simulink model "untitled"  (R2022a)
settings: Solver=FixedStepAuto  StartTime=0.0  StopTime=50  FixedStep=0.0001  RelTol=1e-3
PreLoadFcn:
  | % FK=ss(A,B,C,D);
  | % FK1=tf(FK)
  | G2=tf([-253.6 -141.7 -700.8 2.288],[1 6.083 7.223 17.36 0.6782]);
  | G=G2;
  | figure
  | rlocus(G)
  | rlocfind(G)
  | KP=0.0213;
  | load('peiping.mat');
model workspace: external: MAT-File D:\Desktop\无人机双环pid\peiping.mat (data not in the file)
values from neighbouring files (symbols this model uses):
  A = [0 0 0 0 9.794 0 0 -3.5879 0 0 0 0 ... (144 elements, 12x12)]    [peiping.mat]
  B = [0 0 0 0.0146 0 -0.271 0 0 0 0 -0.151 0 ... (48 elements, 12x4)]    [peiping.mat]
  C = [0 -2 0 0 0 0 -3.5879 0 0 57.3 0 0 ... (240 elements, 20x12)]    [peiping.mat]
  D = [0 0 0 0 0 0 0 0 0 0 0 0 ... (80 elements, 20x4)]    [peiping.mat]
libraries: slpidlib x9
settings Model: PacingRate=1000  Creator=yuhangmeng  LastModifiedBy=yuhangmeng
settings SolverCC: ZeroCrossAlgorithm=Adaptive
settings DataIOCC: ExternalInput=getinputstruct(op_trim2)  InitialState=getstatestruct(op_trim2)
settings DebuggingCC: IgnoredZcDiagnostic=none

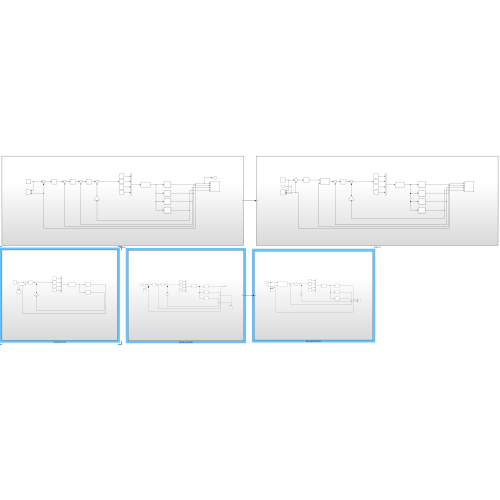
[thumbnail: Simulink's stored preview of the top-level diagram]
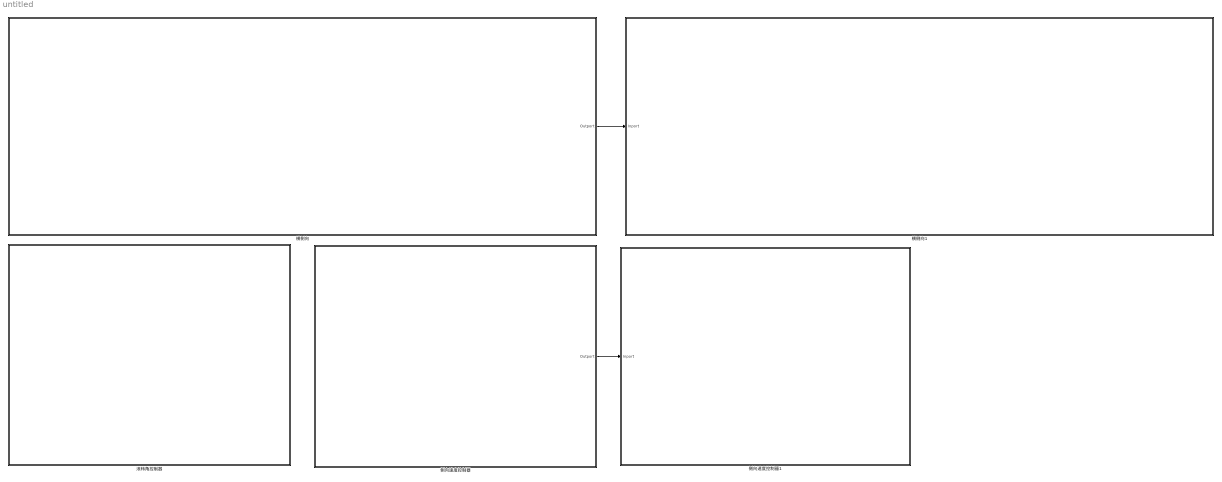
== system untitled ==
  侧向速度控制器 : Subsystem
  侧向速度控制器1 : Subsystem
  横侧向 : Subsystem
  横侧向1 : Subsystem
  滚转角控制器 : Subsystem
  wires:
  侧向速度控制器/1(Outport) -> 侧向速度控制器1/1(Inport)
  横侧向/1(Outport) -> 横侧向1/1(Inport)

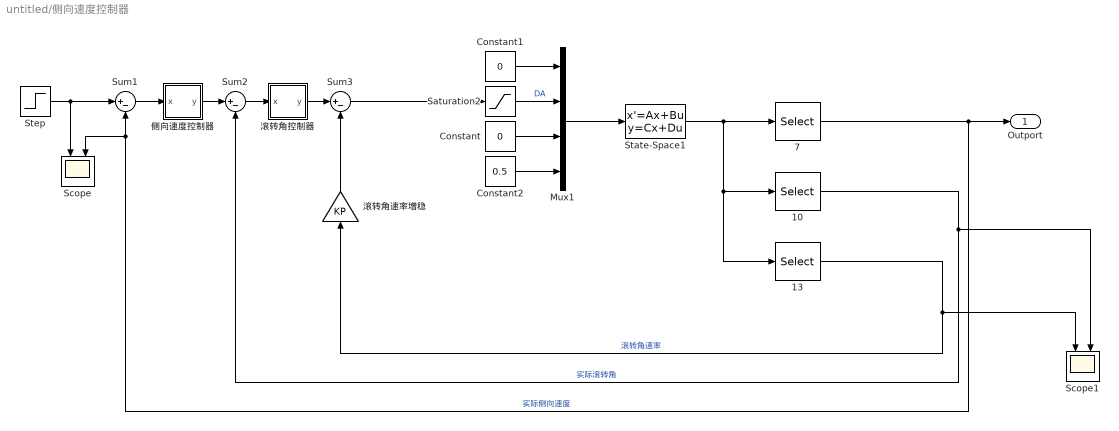
== system untitled/侧向速度控制器 ==
  " 10" : Selector  InputPortWidth=20  IndexOptions=Index vector (dialog)  Indices=10  OutputSizes=1
  " 13" : Selector  InputPortWidth=20  IndexOptions=Index vector (dialog)  Indices=13  OutputSizes=1
  " 7" : Selector  InputPortWidth=20  IndexOptions=Index vector (dialog)  Indices=7  OutputSizes=1
  Constant : Constant  Value=0
  Constant1 : Constant  Value=0
  Constant2 : Constant  Value=0.5
  Mux1 : Mux
  Saturation2 : Saturate  UpperLimit=20  LowerLimit=-20
  Scope : Scope  NumInputPorts=2
  Scope1 : Scope  NumInputPorts=2
  State-Space1 : StateSpace  A=A  B=B  C=C  D=D  InitialCondition=0
  Step : Step  After=10  SampleTime=0
  Sum1 : Sum  Inputs=|+-
  Sum2 : Sum  Inputs=|+-
  Sum3 : Sum  Inputs=|+-
  侧向速度控制器 : Subsystem
  滚转角控制器 : Subsystem
  滚转角速率增稳 : Gain  Gain=KP
  Outport : Outport
  wires:
  Constant/1 -> Mux1/3
  侧向速度控制器/1(y) -> Sum2/1
  Sum2/1 -> 滚转角控制器/1(x)
  Saturation2/1 -> Mux1/2  "DA"
  Sum3/1 -> Saturation2/1
  " 10"/1 -> Scope1/2, Sum2/2  "实际滚转角"
  滚转角控制器/1(y) -> Sum3/1
  " 13"/1 -> Scope1/1, 滚转角速率增稳/1  "滚转角速率"
  State-Space1/1 -> " 13"/1, " 10"/1, " 7"/1
  Constant2/1 -> Mux1/4
  Sum1/1 -> 侧向速度控制器/1(x)
  Mux1/1 -> State-Space1/1
  Constant1/1 -> Mux1/1
  滚转角速率增稳/1 -> Sum3/2
  " 7"/1 -> Scope/2, Sum1/2, Outport/1  "实际侧向速度"
  Step/1 -> Sum1/1, Scope/1

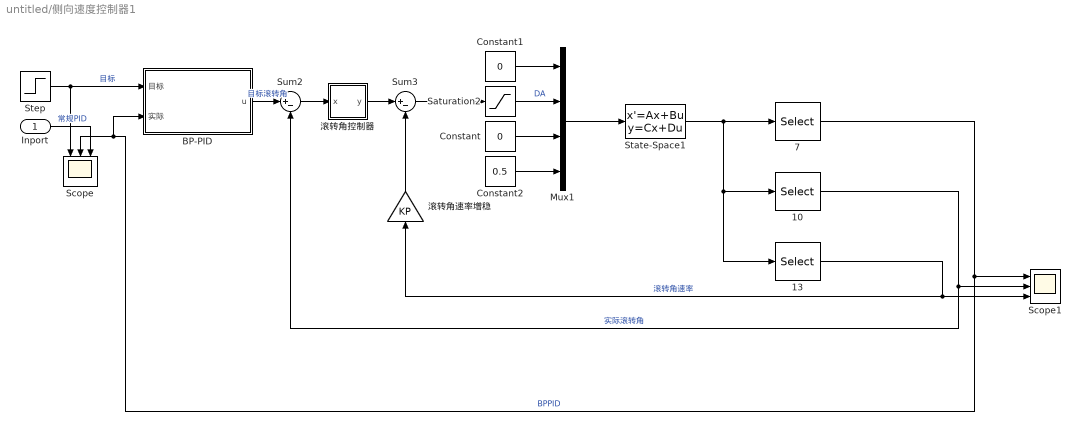
== system untitled/侧向速度控制器1 ==
  Inport : Inport
  " 10" : Selector  InputPortWidth=20  IndexOptions=Index vector (dialog)  Indices=10  OutputSizes=1
  " 13" : Selector  InputPortWidth=20  IndexOptions=Index vector (dialog)  Indices=13  OutputSizes=1
  " 7" : Selector  InputPortWidth=20  IndexOptions=Index vector (dialog)  Indices=7  OutputSizes=1
  BP-PID : Subsystem
  Constant : Constant  Value=0
  Constant1 : Constant  Value=0
  Constant2 : Constant  Value=0.5
  Mux1 : Mux
  Saturation2 : Saturate  UpperLimit=20  LowerLimit=-20
  Scope : Scope  NumInputPorts=3
  Scope1 : Scope  NumInputPorts=3
  State-Space1 : StateSpace  A=A  B=B  C=C  D=D  InitialCondition=0
  Step : Step  Time=0  After=10  SampleTime=0
  Sum2 : Sum  Inputs=|+-
  Sum3 : Sum  Inputs=|+-
  滚转角控制器 : Subsystem
  滚转角速率增稳 : Gain  Gain=KP
  wires:
  Constant/1 -> Mux1/3
  BP-PID/1(u) -> Sum2/1  "目标滚转角"
  Sum2/1 -> 滚转角控制器/1(x)
  Saturation2/1 -> Mux1/2  "DA"
  Sum3/1 -> Saturation2/1
  " 10"/1 -> Scope1/2, Sum2/2  "实际滚转角"
  滚转角控制器/1(y) -> Sum3/1
  " 13"/1 -> Scope1/3, 滚转角速率增稳/1  "滚转角速率"
  State-Space1/1 -> " 13"/1, " 10"/1, " 7"/1
  Constant2/1 -> Mux1/4
  Mux1/1 -> State-Space1/1
  Constant1/1 -> Mux1/1
  滚转角速率增稳/1 -> Sum3/2
  " 7"/1 -> Scope1/1, BP-PID/2(实际), Scope/2  "BPPID"
  Step/1 -> Scope/1, BP-PID/1(目标)  "目标"
  Inport/1 -> Scope/3  "常规PID"

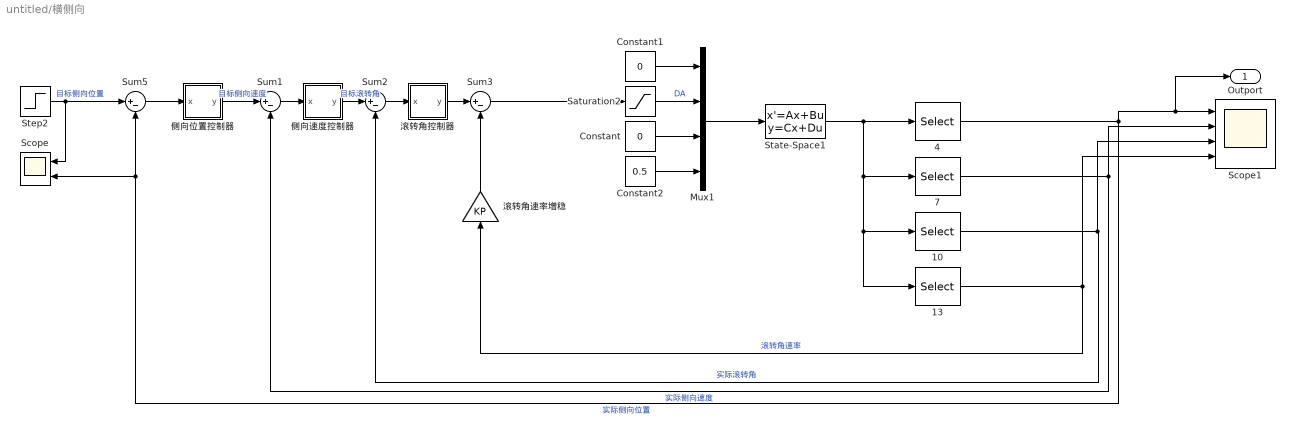
== system untitled/横侧向 ==
  " 10" : Selector  InputPortWidth=20  IndexOptions=Index vector (dialog)  Indices=10  OutputSizes=1
  " 13" : Selector  InputPortWidth=20  IndexOptions=Index vector (dialog)  Indices=13  OutputSizes=1
  " 4" : Selector  InputPortWidth=20  IndexOptions=Index vector (dialog)  Indices=4  OutputSizes=1
  " 7" : Selector  InputPortWidth=20  IndexOptions=Index vector (dialog)  Indices=7  OutputSizes=1
  Constant : Constant  Value=0
  Constant1 : Constant  Value=0
  Constant2 : Constant  Value=0.5
  Mux1 : Mux
  Saturation2 : Saturate  UpperLimit=30  LowerLimit=-30
  Scope : Scope  NumInputPorts=2
  Scope1 : Scope  NumInputPorts=4
  State-Space1 : StateSpace  A=A  B=B  C=C  D=D  InitialCondition=0
  Step2 : Step  Time=0  After=10  SampleTime=0
  Sum{1..3,5} (4 alike) : Sum  Inputs=|+-
  侧向位置控制器 : Subsystem
  侧向速度控制器 : Subsystem
  滚转角控制器 : Subsystem
  滚转角速率增稳 : Gain  Gain=KP
  Outport : Outport
  wires:
  " 4"/1 -> Outport/1, Scope1/1, Sum5/2, Scope/2  "实际侧向位置"
  Constant1/1 -> Mux1/1
  Mux1/1 -> State-Space1/1
  " 7"/1 -> Scope1/2, Sum1/2  "实际侧向速度"
  侧向位置控制器/1(y) -> Sum1/1  "目标侧向速度"
  Sum1/1 -> 侧向速度控制器/1(x)
  " 13"/1 -> 滚转角速率增稳/1, Scope1/4  "滚转角速率"
  Step2/1 -> Scope/1, Sum5/1  "目标侧向位置"
  滚转角控制器/1(y) -> Sum3/1
  State-Space1/1 -> " 10"/1, " 13"/1, " 7"/1, " 4"/1
  " 10"/1 -> Scope1/3, Sum2/2  "实际滚转角"
  Sum5/1 -> 侧向位置控制器/1(x)
  Sum2/1 -> 滚转角控制器/1(x)
  Constant2/1 -> Mux1/4
  滚转角速率增稳/1 -> Sum3/2
  Sum3/1 -> Saturation2/1
  Saturation2/1 -> Mux1/2  "DA"
  侧向速度控制器/1(y) -> Sum2/1  "目标滚转角"
  Constant/1 -> Mux1/3

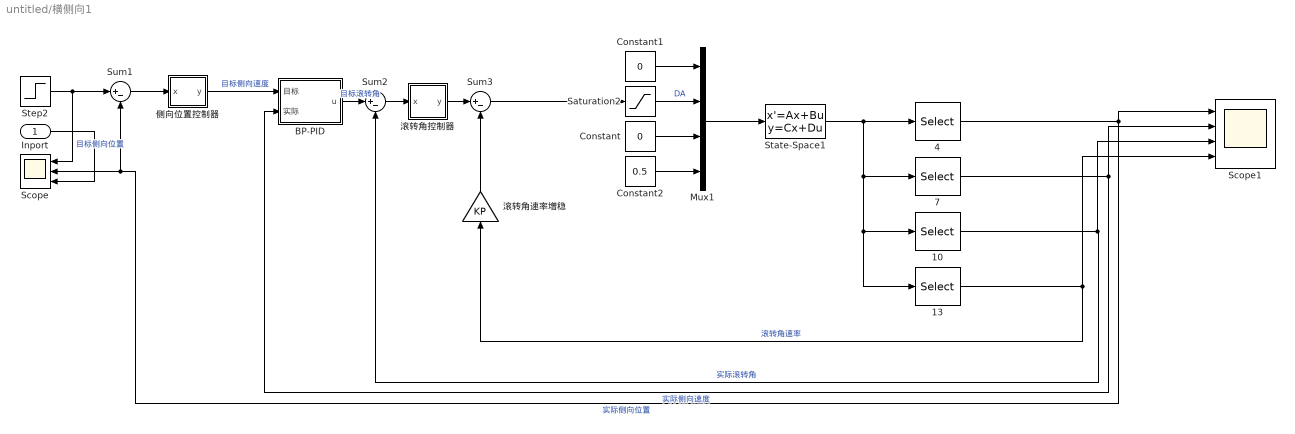
== system untitled/横侧向1 ==
  Inport : Inport
  " 10" : Selector  InputPortWidth=20  IndexOptions=Index vector (dialog)  Indices=10  OutputSizes=1
  " 13" : Selector  InputPortWidth=20  IndexOptions=Index vector (dialog)  Indices=13  OutputSizes=1
  " 4" : Selector  InputPortWidth=20  IndexOptions=Index vector (dialog)  Indices=4  OutputSizes=1
  " 7" : Selector  InputPortWidth=20  IndexOptions=Index vector (dialog)  Indices=7  OutputSizes=1
  BP-PID : Subsystem
  Constant : Constant  Value=0
  Constant1 : Constant  Value=0
  Constant2 : Constant  Value=0.5
  Mux1 : Mux
  Saturation2 : Saturate  UpperLimit=30  LowerLimit=-30
  Scope : Scope  NumInputPorts=3
  Scope1 : Scope  NumInputPorts=4
  State-Space1 : StateSpace  A=A  B=B  C=C  D=D  InitialCondition=0
  Step2 : Step  Time=0  After=10  SampleTime=0
  Sum1 : Sum  Inputs=|+-
  Sum2 : Sum  Inputs=|+-
  Sum3 : Sum  Inputs=|+-
  侧向位置控制器 : Subsystem
  滚转角控制器 : Subsystem
  滚转角速率增稳 : Gain  Gain=KP
  wires:
  " 4"/1 -> Scope1/1, Scope/2, Sum1/2  "实际侧向位置"
  Constant1/1 -> Mux1/1
  Mux1/1 -> State-Space1/1
  " 7"/1 -> BP-PID/2(实际), Scope1/2  "实际侧向速度"
  侧向位置控制器/1(y) -> BP-PID/1(目标)  "目标侧向速度"
  " 13"/1 -> 滚转角速率增稳/1, Scope1/4  "滚转角速率"
  Step2/1 -> Sum1/1, Scope/1  "目标侧向位置"
  滚转角控制器/1(y) -> Sum3/1
  State-Space1/1 -> " 10"/1, " 13"/1, " 7"/1, " 4"/1
  " 10"/1 -> Scope1/3, Sum2/2  "实际滚转角"
  Sum2/1 -> 滚转角控制器/1(x)
  Constant2/1 -> Mux1/4
  滚转角速率增稳/1 -> Sum3/2
  Sum3/1 -> Saturation2/1
  Saturation2/1 -> Mux1/2  "DA"
  BP-PID/1(u) -> Sum2/1  "目标滚转角"
  Constant/1 -> Mux1/3
  Inport/1 -> Scope/3
  Sum1/1 -> 侧向位置控制器/1(x)

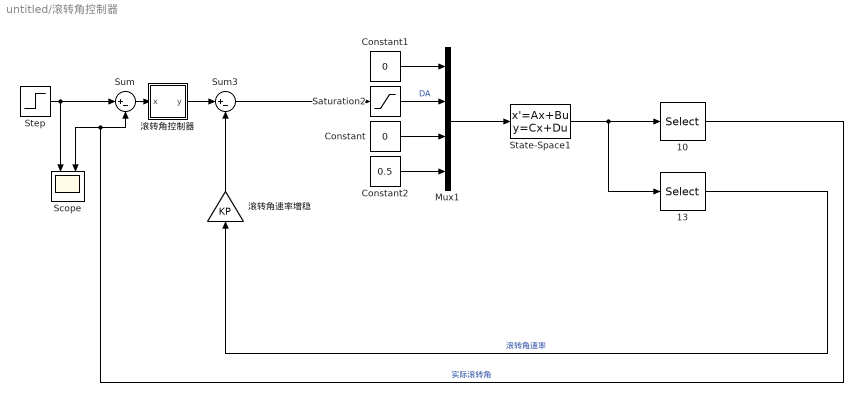
== system untitled/滚转角控制器 ==
  " 10" : Selector  InputPortWidth=20  IndexOptions=Index vector (dialog)  Indices=10  OutputSizes=1
  " 13" : Selector  InputPortWidth=20  IndexOptions=Index vector (dialog)  Indices=13  OutputSizes=1
  Constant : Constant  Value=0
  Constant1 : Constant  Value=0
  Constant2 : Constant  Value=0.5
  Mux1 : Mux
  Saturation2 : Saturate  UpperLimit=20  LowerLimit=-20
  Scope : Scope  NumInputPorts=2
  State-Space1 : StateSpace  A=A  B=B  C=C  D=D  InitialCondition=0
  Step : Step  After=10  SampleTime=0
  Sum : Sum  Inputs=|+-
  Sum3 : Sum  Inputs=|+-
  滚转角控制器 : Subsystem
  滚转角速率增稳 : Gain  Gain=KP
  wires:
  Step/1 -> Sum/1, Scope/1
  " 13"/1 -> 滚转角速率增稳/1  "滚转角速率"
  State-Space1/1 -> " 13"/1, " 10"/1
  Saturation2/1 -> Mux1/2  "DA"
  滚转角控制器/1(y) -> Sum3/1
  Constant/1 -> Mux1/3
  Sum3/1 -> Saturation2/1
  " 10"/1 -> Sum/2, Scope/2  "实际滚转角"
  Constant2/1 -> Mux1/4
  Mux1/1 -> State-Space1/1
  Constant1/1 -> Mux1/1
  滚转角速率增稳/1 -> Sum3/2
  Sum/1 -> 滚转角控制器/1(x)

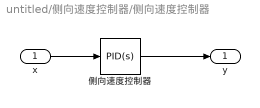
== system untitled/侧向速度控制器/侧向速度控制器 ==
  x : Inport
  侧向速度控制器 : slpidlib/PID Controller  Controller=PID  Form=Parallel  TimeDomain=Continuous-time  UseExternalTs=off  SampleTime=-1  IntegratorMethod=Forward Euler  FilterMethod=Forward Euler  ControllerParametersSource=internal  P=5.34227006077093  I=0.349672749847969  UseKiTs=off  D=2.80119106612119  N=1.85105755121857  UseFilter=on  TunerSelectOption=Transfer Function Based (PID Tuner App)  InitialConditionSource=internal  InitialConditionForIntegrator=0  InitialConditionForFilter=0  DifferentiatorICPrevScaledInput=0  ExternalReset=none  TrackingMode=off  Kt=1  LimitOutput=off  SatLimitsSource=internal  UpperSaturationLimit=inf  LowerSaturationLimit=-inf  LinearizeAsGain=on  AntiWindupMode=none  Kb=1  POutMin=[]  POutMax=[]  IOutMin=[]  IOutMax=[]  DOutMin=[]  DOutMax=[]  NOutMin=[]  NOutMax=[]  SumOutMin=[]  SumOutMax=[]  SaturationOutMin=[]  SaturationOutMax=[]  PParamMin=[]  PParamMax=[]  IParamMin=[]  IParamMax=[]  DParamMin=[]  DParamMax=[]  NParamMin=[]  NParamMax=[]  KbParamMin=[]  KbParamMax=[]  KtParamMin=[]  KtParamMax=[]  KbOutMin=[]  KbOutMax=[]  KtOutMin=[]  KtOutMax=[]  IntegratorOutMin=[]  IntegratorOutMax=[]  FilterOutMin=[]  FilterOutMax=[]  SumI1OutMin=[]  SumI1OutMax=[]  SumI2OutMin=[]  SumI2OutMax=[]  SumI3OutMin=[]  SumI3OutMax=[]  SumI4OutMin=[]  SumI4OutMax=[]  SumDOutMin=[]  SumDOutMax=[]  DifferentiatorOutMin=[]  DifferentiatorOutMax=[]  FilterDiffOutCoefMin=[]  FilterDiffOutCoefMax=[]  ReciprocalOutMin=[]  ReciprocalOutMax=[]  SumDenOutMin=[]  SumDenOutMax=[]  SumNumOutMin=[]  SumNumOutMax=[]  DivideOutMin=[]  DivideOutMax=[]  UdiffTsProdOutMin=[]  UdiffTsProdOutMax=[]  NTsProdOutMin=[]  NTsProdOutMax=[]  UintegralTsProdOutMin=[]  UintegralTsProdOutMax=[]  UngainTsProdOutMin=[]  UngainTsProdOutMax=[]  IntegratorContinuousStateAttributes=''  IntegratorStateMustResolveToSignalObject=off  IntegratorRTWStateStorageClass=Auto  FilterContinuousStateAttributes=''  FilterStateMustResolveToSignalObject=off  FilterRTWStateStorageClass=Auto  ParallelPVariant=InternalParameters  IdealPVariant=Disabled  IVariant=InternalParameters  DVariant=InternalParameters  IntegratorVariant=Continuous  SatVariant=Disabled  AWVariant=Passthrough  PCopyVariant=Disabled  TRVariant=Disabled  FdbkBlocksVariant=Forward  IdealPFdbkVariant=Disabled  SatFdbkVariant=Disabled  DerivativeFilterVariant=ContFilter  NVariant=InternalParameters  NCopyVariant=Disabled  FilterICVariant=InternalICsFilter  IntegratorICVariant=InternalICs  ExternalResetVariant=Disabled  TRSumVariant=Passthrough  SumFdbkVariant=Disabled  SumVariant=Sum_PID  TsampFilterVariant=InternalTs  TsampNgainVariant=Passthrough  TsampIntegralVariant=Passthrough  ExternalSaturationOutDataTypeStr=Inherit: Same as second input  aMode=0
  y : Outport  VectorParamsAs1DForOutWhenUnconnected=off
  wires:
  侧向速度控制器/1 -> y/1
  x/1 -> 侧向速度控制器/1

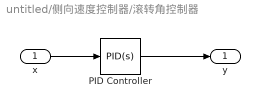
== system untitled/侧向速度控制器/滚转角控制器 ==
  x : Inport
  PID Controller : slpidlib/PID Controller  Controller=PID  Form=Parallel  TimeDomain=Continuous-time  UseExternalTs=off  SampleTime=-1  IntegratorMethod=Forward Euler  FilterMethod=Forward Euler  ControllerParametersSource=internal  P=-26.8091227267229  I=-0.500000001899811  UseKiTs=off  D=-14.2502619165409  N=4974.03399819071  UseFilter=on  TunerSelectOption=Transfer Function Based (PID Tuner App)  InitialConditionSource=internal  InitialConditionForIntegrator=0  InitialConditionForFilter=0  DifferentiatorICPrevScaledInput=0  ExternalReset=none  TrackingMode=off  Kt=1  LimitOutput=off  SatLimitsSource=internal  UpperSaturationLimit=inf  LowerSaturationLimit=-inf  LinearizeAsGain=on  AntiWindupMode=none  Kb=1  POutMin=[]  POutMax=[]  IOutMin=[]  IOutMax=[]  DOutMin=[]  DOutMax=[]  NOutMin=[]  NOutMax=[]  SumOutMin=[]  SumOutMax=[]  SaturationOutMin=[]  SaturationOutMax=[]  PParamMin=[]  PParamMax=[]  IParamMin=[]  IParamMax=[]  DParamMin=[]  DParamMax=[]  NParamMin=[]  NParamMax=[]  KbParamMin=[]  KbParamMax=[]  KtParamMin=[]  KtParamMax=[]  KbOutMin=[]  KbOutMax=[]  KtOutMin=[]  KtOutMax=[]  IntegratorOutMin=[]  IntegratorOutMax=[]  FilterOutMin=[]  FilterOutMax=[]  SumI1OutMin=[]  SumI1OutMax=[]  SumI2OutMin=[]  SumI2OutMax=[]  SumI3OutMin=[]  SumI3OutMax=[]  SumI4OutMin=[]  SumI4OutMax=[]  SumDOutMin=[]  SumDOutMax=[]  DifferentiatorOutMin=[]  DifferentiatorOutMax=[]  FilterDiffOutCoefMin=[]  FilterDiffOutCoefMax=[]  ReciprocalOutMin=[]  ReciprocalOutMax=[]  SumDenOutMin=[]  SumDenOutMax=[]  SumNumOutMin=[]  SumNumOutMax=[]  DivideOutMin=[]  DivideOutMax=[]  UdiffTsProdOutMin=[]  UdiffTsProdOutMax=[]  NTsProdOutMin=[]  NTsProdOutMax=[]  UintegralTsProdOutMin=[]  UintegralTsProdOutMax=[]  UngainTsProdOutMin=[]  UngainTsProdOutMax=[]  IntegratorContinuousStateAttributes=''  IntegratorStateMustResolveToSignalObject=off  IntegratorRTWStateStorageClass=Auto  FilterContinuousStateAttributes=''  FilterStateMustResolveToSignalObject=off  FilterRTWStateStorageClass=Auto  ParallelPVariant=InternalParameters  IdealPVariant=Disabled  IVariant=InternalParameters  DVariant=InternalParameters  IntegratorVariant=Continuous  SatVariant=Disabled  AWVariant=Passthrough  PCopyVariant=Disabled  TRVariant=Disabled  FdbkBlocksVariant=Forward  IdealPFdbkVariant=Disabled  SatFdbkVariant=Disabled  DerivativeFilterVariant=ContFilter  NVariant=InternalParameters  NCopyVariant=Disabled  FilterICVariant=InternalICsFilter  IntegratorICVariant=InternalICs  ExternalResetVariant=Disabled  TRSumVariant=Passthrough  SumFdbkVariant=Disabled  SumVariant=Sum_PID  TsampFilterVariant=InternalTs  TsampNgainVariant=Passthrough  TsampIntegralVariant=Passthrough  ExternalSaturationOutDataTypeStr=Inherit: Same as second input  aMode=0
  y : Outport  VectorParamsAs1DForOutWhenUnconnected=off
  wires:
  x/1 -> PID Controller/1
  PID Controller/1 -> y/1

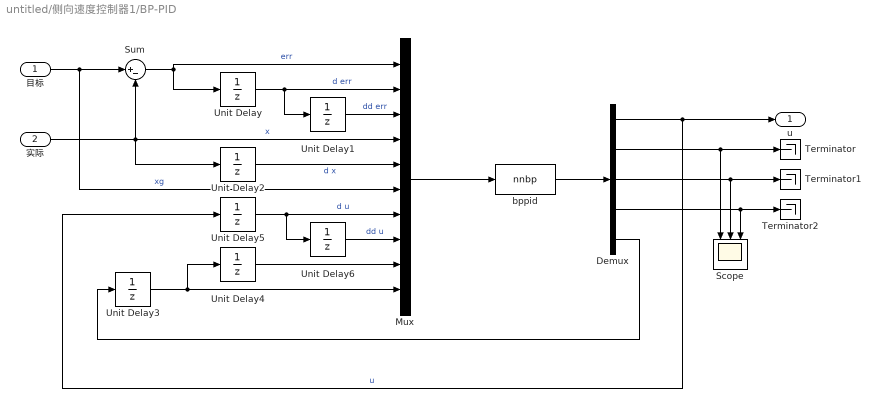
== system untitled/侧向速度控制器1/BP-PID ==
  目标 : Inport
  实际 : Inport  Port=2
  Demux : Demux  Outputs=[1 1 1 1 18]
  Mux : Mux  Inputs=10
  Scope : Scope  NumInputPorts=3
  Sum : Sum  Inputs=|+-
  Terminator : Terminator
  Terminator1 : Terminator
  Terminator2 : Terminator
  Unit Delay{,1..2,4..6} (6 alike) : UnitDelay  SampleTime=-1  HasFrameUpgradeWarning=on
  Unit Delay3 : UnitDelay  InitialCondition=abs(rand(18,1))  SampleTime=-1  HasFrameUpgradeWarning=on
  bppid : S-Function  FunctionName=nnbp  Parameters=nh,xite,alfa  SFunctionDeploymentMode=off  EnableBusSupport=off  mask{nh=3, xite=0.25, alfa=0.25}
      mask prompts: nh "隐含层层数"; xite "学习速率"; alfa "惯性系数"
      mask DialogControl ParameterGroupVar Prompt: 参数
  u : Outport
  wires:
  目标/1 -> Mux/6, Sum/1  "xg"
  实际/1 -> Unit Delay2/1, Sum/2, Mux/4  "x"
  Sum/1 -> Mux/1, Unit Delay/1  "err"
  Unit Delay/1 -> Unit Delay1/1, Mux/2  "d err"
  Unit Delay1/1 -> Mux/3  "dd err"
  Unit Delay2/1 -> Mux/5  "d x"
  Mux/1 -> bppid/1
  bppid/1 -> Demux/1
  Unit Delay3/1 -> Mux/10, Unit Delay4/1
  Unit Delay4/1 -> Mux/9
  Unit Delay5/1 -> Unit Delay6/1, Mux/7  "d u"
  Demux/2 -> Scope/1, Terminator/1
  Demux/3 -> Scope/2, Terminator1/1
  Demux/4 -> Scope/3, Terminator2/1
  Unit Delay6/1 -> Mux/8  "dd u"
  Demux/5 -> Unit Delay3/1
  Demux/1 -> Unit Delay5/1, u/1  "u"

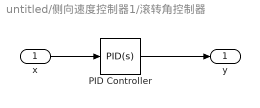
== system untitled/侧向速度控制器1/滚转角控制器 ==
  x : Inport
  PID Controller : slpidlib/PID Controller  Controller=PID  Form=Parallel  TimeDomain=Continuous-time  UseExternalTs=off  SampleTime=-1  IntegratorMethod=Forward Euler  FilterMethod=Forward Euler  ControllerParametersSource=internal  P=-26.8091227267229  I=-0.500000001899811  UseKiTs=off  D=-14.2502619165409  N=4974.03399819071  UseFilter=on  TunerSelectOption=Transfer Function Based (PID Tuner App)  InitialConditionSource=internal  InitialConditionForIntegrator=0  InitialConditionForFilter=0  DifferentiatorICPrevScaledInput=0  ExternalReset=none  TrackingMode=off  Kt=1  LimitOutput=off  SatLimitsSource=internal  UpperSaturationLimit=inf  LowerSaturationLimit=-inf  LinearizeAsGain=on  AntiWindupMode=none  Kb=1  POutMin=[]  POutMax=[]  IOutMin=[]  IOutMax=[]  DOutMin=[]  DOutMax=[]  NOutMin=[]  NOutMax=[]  SumOutMin=[]  SumOutMax=[]  SaturationOutMin=[]  SaturationOutMax=[]  PParamMin=[]  PParamMax=[]  IParamMin=[]  IParamMax=[]  DParamMin=[]  DParamMax=[]  NParamMin=[]  NParamMax=[]  KbParamMin=[]  KbParamMax=[]  KtParamMin=[]  KtParamMax=[]  KbOutMin=[]  KbOutMax=[]  KtOutMin=[]  KtOutMax=[]  IntegratorOutMin=[]  IntegratorOutMax=[]  FilterOutMin=[]  FilterOutMax=[]  SumI1OutMin=[]  SumI1OutMax=[]  SumI2OutMin=[]  SumI2OutMax=[]  SumI3OutMin=[]  SumI3OutMax=[]  SumI4OutMin=[]  SumI4OutMax=[]  SumDOutMin=[]  SumDOutMax=[]  DifferentiatorOutMin=[]  DifferentiatorOutMax=[]  FilterDiffOutCoefMin=[]  FilterDiffOutCoefMax=[]  ReciprocalOutMin=[]  ReciprocalOutMax=[]  SumDenOutMin=[]  SumDenOutMax=[]  SumNumOutMin=[]  SumNumOutMax=[]  DivideOutMin=[]  DivideOutMax=[]  UdiffTsProdOutMin=[]  UdiffTsProdOutMax=[]  NTsProdOutMin=[]  NTsProdOutMax=[]  UintegralTsProdOutMin=[]  UintegralTsProdOutMax=[]  UngainTsProdOutMin=[]  UngainTsProdOutMax=[]  IntegratorContinuousStateAttributes=''  IntegratorStateMustResolveToSignalObject=off  IntegratorRTWStateStorageClass=Auto  FilterContinuousStateAttributes=''  FilterStateMustResolveToSignalObject=off  FilterRTWStateStorageClass=Auto  ParallelPVariant=InternalParameters  IdealPVariant=Disabled  IVariant=InternalParameters  DVariant=InternalParameters  IntegratorVariant=Continuous  SatVariant=Disabled  AWVariant=Passthrough  PCopyVariant=Disabled  TRVariant=Disabled  FdbkBlocksVariant=Forward  IdealPFdbkVariant=Disabled  SatFdbkVariant=Disabled  DerivativeFilterVariant=ContFilter  NVariant=InternalParameters  NCopyVariant=Disabled  FilterICVariant=InternalICsFilter  IntegratorICVariant=InternalICs  ExternalResetVariant=Disabled  TRSumVariant=Passthrough  SumFdbkVariant=Disabled  SumVariant=Sum_PID  TsampFilterVariant=InternalTs  TsampNgainVariant=Passthrough  TsampIntegralVariant=Passthrough  ExternalSaturationOutDataTypeStr=Inherit: Same as second input  aMode=0
  y : Outport  VectorParamsAs1DForOutWhenUnconnected=off
  wires:
  x/1 -> PID Controller/1
  PID Controller/1 -> y/1

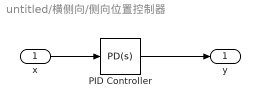
== system untitled/横侧向/侧向位置控制器 ==
  x : Inport
  PID Controller : slpidlib/PID Controller  Controller=PD  Form=Parallel  TimeDomain=Continuous-time  UseExternalTs=off  SampleTime=-1  IntegratorMethod=Forward Euler  FilterMethod=Forward Euler  ControllerParametersSource=internal  P=0.14  I=0  UseKiTs=off  D=0  N=100  UseFilter=on  TunerSelectOption=Transfer Function Based (PID Tuner App)  InitialConditionSource=internal  InitialConditionForIntegrator=0  InitialConditionForFilter=0  DifferentiatorICPrevScaledInput=0  ExternalReset=none  TrackingMode=off  Kt=1  LimitOutput=off  SatLimitsSource=internal  UpperSaturationLimit=inf  LowerSaturationLimit=-inf  LinearizeAsGain=on  AntiWindupMode=none  Kb=1  POutMin=[]  POutMax=[]  IOutMin=[]  IOutMax=[]  DOutMin=[]  DOutMax=[]  NOutMin=[]  NOutMax=[]  SumOutMin=[]  SumOutMax=[]  SaturationOutMin=[]  SaturationOutMax=[]  PParamMin=[]  PParamMax=[]  IParamMin=[]  IParamMax=[]  DParamMin=[]  DParamMax=[]  NParamMin=[]  NParamMax=[]  KbParamMin=[]  KbParamMax=[]  KtParamMin=[]  KtParamMax=[]  KbOutMin=[]  KbOutMax=[]  KtOutMin=[]  KtOutMax=[]  IntegratorOutMin=[]  IntegratorOutMax=[]  FilterOutMin=[]  FilterOutMax=[]  SumI1OutMin=[]  SumI1OutMax=[]  SumI2OutMin=[]  SumI2OutMax=[]  SumI3OutMin=[]  SumI3OutMax=[]  SumI4OutMin=[]  SumI4OutMax=[]  SumDOutMin=[]  SumDOutMax=[]  DifferentiatorOutMin=[]  DifferentiatorOutMax=[]  FilterDiffOutCoefMin=[]  FilterDiffOutCoefMax=[]  ReciprocalOutMin=[]  ReciprocalOutMax=[]  SumDenOutMin=[]  SumDenOutMax=[]  SumNumOutMin=[]  SumNumOutMax=[]  DivideOutMin=[]  DivideOutMax=[]  UdiffTsProdOutMin=[]  UdiffTsProdOutMax=[]  NTsProdOutMin=[]  NTsProdOutMax=[]  UintegralTsProdOutMin=[]  UintegralTsProdOutMax=[]  UngainTsProdOutMin=[]  UngainTsProdOutMax=[]  IntegratorContinuousStateAttributes=''  IntegratorStateMustResolveToSignalObject=off  IntegratorRTWStateStorageClass=Auto  FilterContinuousStateAttributes=''  FilterStateMustResolveToSignalObject=off  FilterRTWStateStorageClass=Auto  ParallelPVariant=InternalParameters  IdealPVariant=Disabled  IVariant=Disabled  DVariant=InternalParameters  IntegratorVariant=Disabled  SatVariant=Disabled  AWVariant=Disabled  PCopyVariant=Disabled  TRVariant=Disabled  FdbkBlocksVariant=Forward  IdealPFdbkVariant=Disabled  SatFdbkVariant=Disabled  DerivativeFilterVariant=ContFilter  NVariant=InternalParameters  NCopyVariant=Disabled  FilterICVariant=InternalICsFilter  IntegratorICVariant=Disabled  ExternalResetVariant=Disabled  TRSumVariant=Passthrough  SumFdbkVariant=Disabled  SumVariant=Sum_PD  TsampFilterVariant=InternalTs  TsampNgainVariant=Passthrough  TsampIntegralVariant=Disabled_SignalSpec  ExternalSaturationOutDataTypeStr=Inherit: Same as second input  aMode=0
  y : Outport  VectorParamsAs1DForOutWhenUnconnected=off
  wires:
  x/1 -> PID Controller/1
  PID Controller/1 -> y/1

== system untitled/横侧向/侧向速度控制器 ==
  x : Inport
  侧向速度控制器 : slpidlib/PID Controller  Controller=PID  Form=Parallel  TimeDomain=Continuous-time  UseExternalTs=off  SampleTime=-1  IntegratorMethod=Forward Euler  FilterMethod=Forward Euler  ControllerParametersSource=internal  P=5.34227006077093  I=0.349672749847969  UseKiTs=off  D=2.80119106612119  N=1.85105755121857  UseFilter=on  TunerSelectOption=Transfer Function Based (PID Tuner App)  InitialConditionSource=internal  InitialConditionForIntegrator=0  InitialConditionForFilter=0  DifferentiatorICPrevScaledInput=0  ExternalReset=none  TrackingMode=off  Kt=1  LimitOutput=off  SatLimitsSource=internal  UpperSaturationLimit=inf  LowerSaturationLimit=-inf  LinearizeAsGain=on  AntiWindupMode=none  Kb=1  POutMin=[]  POutMax=[]  IOutMin=[]  IOutMax=[]  DOutMin=[]  DOutMax=[]  NOutMin=[]  NOutMax=[]  SumOutMin=[]  SumOutMax=[]  SaturationOutMin=[]  SaturationOutMax=[]  PParamMin=[]  PParamMax=[]  IParamMin=[]  IParamMax=[]  DParamMin=[]  DParamMax=[]  NParamMin=[]  NParamMax=[]  KbParamMin=[]  KbParamMax=[]  KtParamMin=[]  KtParamMax=[]  KbOutMin=[]  KbOutMax=[]  KtOutMin=[]  KtOutMax=[]  IntegratorOutMin=[]  IntegratorOutMax=[]  FilterOutMin=[]  FilterOutMax=[]  SumI1OutMin=[]  SumI1OutMax=[]  SumI2OutMin=[]  SumI2OutMax=[]  SumI3OutMin=[]  SumI3OutMax=[]  SumI4OutMin=[]  SumI4OutMax=[]  SumDOutMin=[]  SumDOutMax=[]  DifferentiatorOutMin=[]  DifferentiatorOutMax=[]  FilterDiffOutCoefMin=[]  FilterDiffOutCoefMax=[]  ReciprocalOutMin=[]  ReciprocalOutMax=[]  SumDenOutMin=[]  SumDenOutMax=[]  SumNumOutMin=[]  SumNumOutMax=[]  DivideOutMin=[]  DivideOutMax=[]  UdiffTsProdOutMin=[]  UdiffTsProdOutMax=[]  NTsProdOutMin=[]  NTsProdOutMax=[]  UintegralTsProdOutMin=[]  UintegralTsProdOutMax=[]  UngainTsProdOutMin=[]  UngainTsProdOutMax=[]  IntegratorContinuousStateAttributes=''  IntegratorStateMustResolveToSignalObject=off  IntegratorRTWStateStorageClass=Auto  FilterContinuousStateAttributes=''  FilterStateMustResolveToSignalObject=off  FilterRTWStateStorageClass=Auto  ParallelPVariant=InternalParameters  IdealPVariant=Disabled  IVariant=InternalParameters  DVariant=InternalParameters  IntegratorVariant=Continuous  SatVariant=Disabled  AWVariant=Passthrough  PCopyVariant=Disabled  TRVariant=Disabled  FdbkBlocksVariant=Forward  IdealPFdbkVariant=Disabled  SatFdbkVariant=Disabled  DerivativeFilterVariant=ContFilter  NVariant=InternalParameters  NCopyVariant=Disabled  FilterICVariant=InternalICsFilter  IntegratorICVariant=InternalICs  ExternalResetVariant=Disabled  TRSumVariant=Passthrough  SumFdbkVariant=Disabled  SumVariant=Sum_PID  TsampFilterVariant=InternalTs  TsampNgainVariant=Passthrough  TsampIntegralVariant=Passthrough  ExternalSaturationOutDataTypeStr=Inherit: Same as second input  aMode=0
  y : Outport  VectorParamsAs1DForOutWhenUnconnected=off
  wires:
  侧向速度控制器/1 -> y/1
  x/1 -> 侧向速度控制器/1

== system untitled/横侧向/滚转角控制器 ==
  x : Inport
  PID Controller : slpidlib/PID Controller  Controller=PID  Form=Parallel  TimeDomain=Continuous-time  UseExternalTs=off  SampleTime=-1  IntegratorMethod=Forward Euler  FilterMethod=Forward Euler  ControllerParametersSource=internal  P=-26.8091227267229  I=-0.500000001899811  UseKiTs=off  D=-14.2502619165409  N=4974.03399819071  UseFilter=on  TunerSelectOption=Transfer Function Based (PID Tuner App)  InitialConditionSource=internal  InitialConditionForIntegrator=0  InitialConditionForFilter=0  DifferentiatorICPrevScaledInput=0  ExternalReset=none  TrackingMode=off  Kt=1  LimitOutput=off  SatLimitsSource=internal  UpperSaturationLimit=inf  LowerSaturationLimit=-inf  LinearizeAsGain=on  AntiWindupMode=none  Kb=1  POutMin=[]  POutMax=[]  IOutMin=[]  IOutMax=[]  DOutMin=[]  DOutMax=[]  NOutMin=[]  NOutMax=[]  SumOutMin=[]  SumOutMax=[]  SaturationOutMin=[]  SaturationOutMax=[]  PParamMin=[]  PParamMax=[]  IParamMin=[]  IParamMax=[]  DParamMin=[]  DParamMax=[]  NParamMin=[]  NParamMax=[]  KbParamMin=[]  KbParamMax=[]  KtParamMin=[]  KtParamMax=[]  KbOutMin=[]  KbOutMax=[]  KtOutMin=[]  KtOutMax=[]  IntegratorOutMin=[]  IntegratorOutMax=[]  FilterOutMin=[]  FilterOutMax=[]  SumI1OutMin=[]  SumI1OutMax=[]  SumI2OutMin=[]  SumI2OutMax=[]  SumI3OutMin=[]  SumI3OutMax=[]  SumI4OutMin=[]  SumI4OutMax=[]  SumDOutMin=[]  SumDOutMax=[]  DifferentiatorOutMin=[]  DifferentiatorOutMax=[]  FilterDiffOutCoefMin=[]  FilterDiffOutCoefMax=[]  ReciprocalOutMin=[]  ReciprocalOutMax=[]  SumDenOutMin=[]  SumDenOutMax=[]  SumNumOutMin=[]  SumNumOutMax=[]  DivideOutMin=[]  DivideOutMax=[]  UdiffTsProdOutMin=[]  UdiffTsProdOutMax=[]  NTsProdOutMin=[]  NTsProdOutMax=[]  UintegralTsProdOutMin=[]  UintegralTsProdOutMax=[]  UngainTsProdOutMin=[]  UngainTsProdOutMax=[]  IntegratorContinuousStateAttributes=''  IntegratorStateMustResolveToSignalObject=off  IntegratorRTWStateStorageClass=Auto  FilterContinuousStateAttributes=''  FilterStateMustResolveToSignalObject=off  FilterRTWStateStorageClass=Auto  ParallelPVariant=InternalParameters  IdealPVariant=Disabled  IVariant=InternalParameters  DVariant=InternalParameters  IntegratorVariant=Continuous  SatVariant=Disabled  AWVariant=Passthrough  PCopyVariant=Disabled  TRVariant=Disabled  FdbkBlocksVariant=Forward  IdealPFdbkVariant=Disabled  SatFdbkVariant=Disabled  DerivativeFilterVariant=ContFilter  NVariant=InternalParameters  NCopyVariant=Disabled  FilterICVariant=InternalICsFilter  IntegratorICVariant=InternalICs  ExternalResetVariant=Disabled  TRSumVariant=Passthrough  SumFdbkVariant=Disabled  SumVariant=Sum_PID  TsampFilterVariant=InternalTs  TsampNgainVariant=Passthrough  TsampIntegralVariant=Passthrough  ExternalSaturationOutDataTypeStr=Inherit: Same as second input  aMode=0
  y : Outport  VectorParamsAs1DForOutWhenUnconnected=off
  wires:
  x/1 -> PID Controller/1
  PID Controller/1 -> y/1

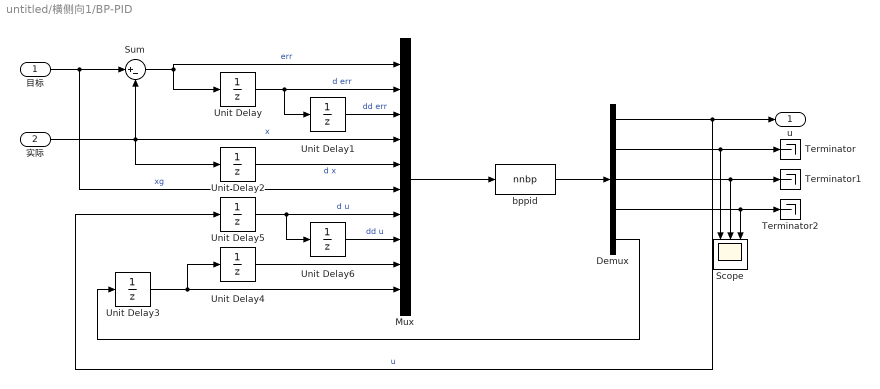
== system untitled/横侧向1/BP-PID ==
  目标 : Inport
  实际 : Inport  Port=2
  Demux : Demux  Outputs=[1 1 1 1 18]
  Mux : Mux  Inputs=10
  Scope : Scope  NumInputPorts=3
  Sum : Sum  Inputs=|+-
  Terminator : Terminator
  Terminator1 : Terminator
  Terminator2 : Terminator
  Unit Delay{,1..2,4..6} (6 alike) : UnitDelay  SampleTime=-1  HasFrameUpgradeWarning=on
  Unit Delay3 : UnitDelay  InitialCondition=abs(rand(18,1))  SampleTime=-1  HasFrameUpgradeWarning=on
  bppid : S-Function  FunctionName=nnbp  Parameters=nh,xite,alfa  SFunctionDeploymentMode=off  EnableBusSupport=off  mask{nh=3, xite=0.25, alfa=0.25}
      mask prompts: nh "隐含层层数"; xite "学习速率"; alfa "惯性系数"
      mask DialogControl ParameterGroupVar Prompt: 参数
  u : Outport
  wires:
  Demux/5 -> Unit Delay3/1
  Unit Delay6/1 -> Mux/8  "dd u"
  Demux/4 -> Scope/3, Terminator2/1
  Demux/3 -> Scope/2, Terminator1/1
  Demux/2 -> Scope/1, Terminator/1
  Unit Delay5/1 -> Mux/7, Unit Delay6/1  "d u"
  Unit Delay4/1 -> Mux/9
  Unit Delay3/1 -> Unit Delay4/1, Mux/10
  bppid/1 -> Demux/1
  Mux/1 -> bppid/1
  Unit Delay2/1 -> Mux/5  "d x"
  Unit Delay1/1 -> Mux/3  "dd err"
  Unit Delay/1 -> Mux/2, Unit Delay1/1  "d err"
  Sum/1 -> Unit Delay/1, Mux/1  "err"
  实际/1 -> Mux/4, Sum/2, Unit Delay2/1  "x"
  Demux/1 -> Unit Delay5/1, u/1  "u"
  目标/1 -> Sum/1, Mux/6  "xg"

== system untitled/横侧向1/侧向位置控制器 ==
  x : Inport
  PID Controller : slpidlib/PID Controller  Controller=PID  Form=Parallel  TimeDomain=Continuous-time  UseExternalTs=off  SampleTime=-1  IntegratorMethod=Forward Euler  FilterMethod=Forward Euler  ControllerParametersSource=internal  P=0.1  I=0  UseKiTs=off  D=0.1  N=100  UseFilter=on  TunerSelectOption=Transfer Function Based (PID Tuner App)  InitialConditionSource=internal  InitialConditionForIntegrator=0  InitialConditionForFilter=0  DifferentiatorICPrevScaledInput=0  ExternalReset=none  TrackingMode=off  Kt=1  LimitOutput=off  SatLimitsSource=internal  UpperSaturationLimit=inf  LowerSaturationLimit=-inf  LinearizeAsGain=on  AntiWindupMode=none  Kb=1  POutMin=[]  POutMax=[]  IOutMin=[]  IOutMax=[]  DOutMin=[]  DOutMax=[]  NOutMin=[]  NOutMax=[]  SumOutMin=[]  SumOutMax=[]  SaturationOutMin=[]  SaturationOutMax=[]  PParamMin=[]  PParamMax=[]  IParamMin=[]  IParamMax=[]  DParamMin=[]  DParamMax=[]  NParamMin=[]  NParamMax=[]  KbParamMin=[]  KbParamMax=[]  KtParamMin=[]  KtParamMax=[]  KbOutMin=[]  KbOutMax=[]  KtOutMin=[]  KtOutMax=[]  IntegratorOutMin=[]  IntegratorOutMax=[]  FilterOutMin=[]  FilterOutMax=[]  SumI1OutMin=[]  SumI1OutMax=[]  SumI2OutMin=[]  SumI2OutMax=[]  SumI3OutMin=[]  SumI3OutMax=[]  SumI4OutMin=[]  SumI4OutMax=[]  SumDOutMin=[]  SumDOutMax=[]  DifferentiatorOutMin=[]  DifferentiatorOutMax=[]  FilterDiffOutCoefMin=[]  FilterDiffOutCoefMax=[]  ReciprocalOutMin=[]  ReciprocalOutMax=[]  SumDenOutMin=[]  SumDenOutMax=[]  SumNumOutMin=[]  SumNumOutMax=[]  DivideOutMin=[]  DivideOutMax=[]  UdiffTsProdOutMin=[]  UdiffTsProdOutMax=[]  NTsProdOutMin=[]  NTsProdOutMax=[]  UintegralTsProdOutMin=[]  UintegralTsProdOutMax=[]  UngainTsProdOutMin=[]  UngainTsProdOutMax=[]  IntegratorContinuousStateAttributes=''  IntegratorStateMustResolveToSignalObject=off  IntegratorRTWStateStorageClass=Auto  FilterContinuousStateAttributes=''  FilterStateMustResolveToSignalObject=off  FilterRTWStateStorageClass=Auto  ParallelPVariant=InternalParameters  IdealPVariant=Disabled  IVariant=InternalParameters  DVariant=InternalParameters  IntegratorVariant=Continuous  SatVariant=Disabled  AWVariant=Passthrough  PCopyVariant=Disabled  TRVariant=Disabled  FdbkBlocksVariant=Forward  IdealPFdbkVariant=Disabled  SatFdbkVariant=Disabled  DerivativeFilterVariant=ContFilter  NVariant=InternalParameters  NCopyVariant=Disabled  FilterICVariant=InternalICsFilter  IntegratorICVariant=InternalICs  ExternalResetVariant=Disabled  TRSumVariant=Passthrough  SumFdbkVariant=Disabled  SumVariant=Sum_PID  TsampFilterVariant=InternalTs  TsampNgainVariant=Passthrough  TsampIntegralVariant=Passthrough  ExternalSaturationOutDataTypeStr=Inherit: Same as second input  aMode=0
  y : Outport  VectorParamsAs1DForOutWhenUnconnected=off
  wires:
  x/1 -> PID Controller/1
  PID Controller/1 -> y/1

== system untitled/横侧向1/滚转角控制器 ==
  x : Inport
  PID Controller : slpidlib/PID Controller  Controller=PID  Form=Parallel  TimeDomain=Continuous-time  UseExternalTs=off  SampleTime=-1  IntegratorMethod=Forward Euler  FilterMethod=Forward Euler  ControllerParametersSource=internal  P=-1.7  I=-0.5  UseKiTs=off  D=-1.7  N=100  UseFilter=on  TunerSelectOption=Transfer Function Based (PID Tuner App)  InitialConditionSource=internal  InitialConditionForIntegrator=0  InitialConditionForFilter=0  DifferentiatorICPrevScaledInput=0  ExternalReset=none  TrackingMode=off  Kt=1  LimitOutput=off  SatLimitsSource=internal  UpperSaturationLimit=inf  LowerSaturationLimit=-inf  LinearizeAsGain=on  AntiWindupMode=none  Kb=1  POutMin=[]  POutMax=[]  IOutMin=[]  IOutMax=[]  DOutMin=[]  DOutMax=[]  NOutMin=[]  NOutMax=[]  SumOutMin=[]  SumOutMax=[]  SaturationOutMin=[]  SaturationOutMax=[]  PParamMin=[]  PParamMax=[]  IParamMin=[]  IParamMax=[]  DParamMin=[]  DParamMax=[]  NParamMin=[]  NParamMax=[]  KbParamMin=[]  KbParamMax=[]  KtParamMin=[]  KtParamMax=[]  KbOutMin=[]  KbOutMax=[]  KtOutMin=[]  KtOutMax=[]  IntegratorOutMin=[]  IntegratorOutMax=[]  FilterOutMin=[]  FilterOutMax=[]  SumI1OutMin=[]  SumI1OutMax=[]  SumI2OutMin=[]  SumI2OutMax=[]  SumI3OutMin=[]  SumI3OutMax=[]  SumI4OutMin=[]  SumI4OutMax=[]  SumDOutMin=[]  SumDOutMax=[]  DifferentiatorOutMin=[]  DifferentiatorOutMax=[]  FilterDiffOutCoefMin=[]  FilterDiffOutCoefMax=[]  ReciprocalOutMin=[]  ReciprocalOutMax=[]  SumDenOutMin=[]  SumDenOutMax=[]  SumNumOutMin=[]  SumNumOutMax=[]  DivideOutMin=[]  DivideOutMax=[]  UdiffTsProdOutMin=[]  UdiffTsProdOutMax=[]  NTsProdOutMin=[]  NTsProdOutMax=[]  UintegralTsProdOutMin=[]  UintegralTsProdOutMax=[]  UngainTsProdOutMin=[]  UngainTsProdOutMax=[]  IntegratorContinuousStateAttributes=''  IntegratorStateMustResolveToSignalObject=off  IntegratorRTWStateStorageClass=Auto  FilterContinuousStateAttributes=''  FilterStateMustResolveToSignalObject=off  FilterRTWStateStorageClass=Auto  ParallelPVariant=InternalParameters  IdealPVariant=Disabled  IVariant=InternalParameters  DVariant=InternalParameters  IntegratorVariant=Continuous  SatVariant=Disabled  AWVariant=Passthrough  PCopyVariant=Disabled  TRVariant=Disabled  FdbkBlocksVariant=Forward  IdealPFdbkVariant=Disabled  SatFdbkVariant=Disabled  DerivativeFilterVariant=ContFilter  NVariant=InternalParameters  NCopyVariant=Disabled  FilterICVariant=InternalICsFilter  IntegratorICVariant=InternalICs  ExternalResetVariant=Disabled  TRSumVariant=Passthrough  SumFdbkVariant=Disabled  SumVariant=Sum_PID  TsampFilterVariant=InternalTs  TsampNgainVariant=Passthrough  TsampIntegralVariant=Passthrough  ExternalSaturationOutDataTypeStr=Inherit: Same as second input  aMode=0
  y : Outport  VectorParamsAs1DForOutWhenUnconnected=off
  wires:
  x/1 -> PID Controller/1
  PID Controller/1 -> y/1

== system untitled/滚转角控制器/滚转角控制器 ==
  x : Inport
  PID Controller : slpidlib/PID Controller  Controller=PID  Form=Parallel  TimeDomain=Continuous-time  UseExternalTs=off  SampleTime=-1  IntegratorMethod=Forward Euler  FilterMethod=Forward Euler  ControllerParametersSource=internal  P=-26.8091227267229  I=-0.500000001899811  UseKiTs=off  D=-14.2502619165409  N=4974.03399819071  UseFilter=on  TunerSelectOption=Transfer Function Based (PID Tuner App)  InitialConditionSource=internal  InitialConditionForIntegrator=0  InitialConditionForFilter=0  DifferentiatorICPrevScaledInput=0  ExternalReset=none  TrackingMode=off  Kt=1  LimitOutput=off  SatLimitsSource=internal  UpperSaturationLimit=inf  LowerSaturationLimit=-inf  LinearizeAsGain=on  AntiWindupMode=none  Kb=1  POutMin=[]  POutMax=[]  IOutMin=[]  IOutMax=[]  DOutMin=[]  DOutMax=[]  NOutMin=[]  NOutMax=[]  SumOutMin=[]  SumOutMax=[]  SaturationOutMin=[]  SaturationOutMax=[]  PParamMin=[]  PParamMax=[]  IParamMin=[]  IParamMax=[]  DParamMin=[]  DParamMax=[]  NParamMin=[]  NParamMax=[]  KbParamMin=[]  KbParamMax=[]  KtParamMin=[]  KtParamMax=[]  KbOutMin=[]  KbOutMax=[]  KtOutMin=[]  KtOutMax=[]  IntegratorOutMin=[]  IntegratorOutMax=[]  FilterOutMin=[]  FilterOutMax=[]  SumI1OutMin=[]  SumI1OutMax=[]  SumI2OutMin=[]  SumI2OutMax=[]  SumI3OutMin=[]  SumI3OutMax=[]  SumI4OutMin=[]  SumI4OutMax=[]  SumDOutMin=[]  SumDOutMax=[]  DifferentiatorOutMin=[]  DifferentiatorOutMax=[]  FilterDiffOutCoefMin=[]  FilterDiffOutCoefMax=[]  ReciprocalOutMin=[]  ReciprocalOutMax=[]  SumDenOutMin=[]  SumDenOutMax=[]  SumNumOutMin=[]  SumNumOutMax=[]  DivideOutMin=[]  DivideOutMax=[]  UdiffTsProdOutMin=[]  UdiffTsProdOutMax=[]  NTsProdOutMin=[]  NTsProdOutMax=[]  UintegralTsProdOutMin=[]  UintegralTsProdOutMax=[]  UngainTsProdOutMin=[]  UngainTsProdOutMax=[]  IntegratorContinuousStateAttributes=''  IntegratorStateMustResolveToSignalObject=off  IntegratorRTWStateStorageClass=Auto  FilterContinuousStateAttributes=''  FilterStateMustResolveToSignalObject=off  FilterRTWStateStorageClass=Auto  ParallelPVariant=InternalParameters  IdealPVariant=Disabled  IVariant=InternalParameters  DVariant=InternalParameters  IntegratorVariant=Continuous  SatVariant=Disabled  AWVariant=Passthrough  PCopyVariant=Disabled  TRVariant=Disabled  FdbkBlocksVariant=Forward  IdealPFdbkVariant=Disabled  SatFdbkVariant=Disabled  DerivativeFilterVariant=ContFilter  NVariant=InternalParameters  NCopyVariant=Disabled  FilterICVariant=InternalICsFilter  IntegratorICVariant=InternalICs  ExternalResetVariant=Disabled  TRSumVariant=Passthrough  SumFdbkVariant=Disabled  SumVariant=Sum_PID  TsampFilterVariant=InternalTs  TsampNgainVariant=Passthrough  TsampIntegralVariant=Passthrough  ExternalSaturationOutDataTypeStr=Inherit: Same as second input  aMode=0
  y : Outport  VectorParamsAs1DForOutWhenUnconnected=off
  wires:
  x/1 -> PID Controller/1
  PID Controller/1 -> y/1
